simulink model "RGBLEDDimmer_model"  (R2024a)
settings: Solver=FixedStepAuto  StartTime=0.0  StopTime=tFinal  FixedStep=T  RelTol=1e-3  EnableMultiTasking=on
libraries: arduinolib x3, simulink x3
settings Model: SimulationMode=external  ExtModeTrigDuration=2  Creator=Christopher  LastModifiedBy=chris
settings SolverCC: AlgebraicLoopSolver=TrustRegion  AutoInsertRateTranBlk=on
settings DataIOCC: LimitDataPoints=on  StreamToWorkspace=on  ReturnWorkspaceOutputs=off
settings OptimizationCC: LifeSpan=1  MaxStackSize=64
settings DebuggingCC: UnconnectedInputMsg=warning  UnconnectedOutputMsg=warning  UnconnectedLineMsg=warning  AllowSymbolicDim=off  SFUnexpectedBacktrackingDiag=warning  SFNoUnconditionalDefaultTransitionDiag=warning  SFExecutionAtInitializationDiag=none  ArithmeticOperatorsInVariantConditions=warning
settings HardwareCC: ProdBitPerInt=16  ProdBitPerPointer=16  ProdBitPerSizeT=16  ProdBitPerPtrDiffT=16  ProdLargestAtomicFloat=None  ProdWordSize=8  ProdHWDeviceType=Atmel->AVR
settings ModelReferenceCC: EnableRefExpFcnMdlSchedulingChecks=on  PropagateSignalLabelsOutOfModel=off
settings SFSimCC: SimUseLocalCustomCode=off  CustomCodeUndefinedFunction=UseInterfaceOnly
settings RTWCC: Description=Embedded Coder  SystemTargetFile=ert.tlc  HardwareBoard=Arduino Nano 3.0  TemplateMakefile=ert_default_tmf  RTWVerbose=off  RTWUseLocalCustomCode=off  Toolchain=Arduino AVR  BuildConfiguration=Faster Runs  GPUComputeCapability=3.5
settings CodeAppCC: MangleLength=10  StateflowObjectComments=on
settings ERTTargetCC: MultiwordLength=2048  ERTCustomFileBanners=off  SupportContinuousTime=on  SupportNonInlinedSFcns=on  RemoveResetFunc=off  SupportVariableSizeSignals=on  ModelStepFunctionPrototypeControlCompliant=off  ExtMode=on  ExtModeTransport=3  ExtModeStaticAlloc=on  ExtModeAutomaticAllocSize=off  ExtModeStaticAllocSize=250  ExtModeMexFile=ext_xcp  ExtModeMexArgs='127.0.0.1' 0 17725  ExtModeIntrfLevel=Level2 - Open  ERTSrcFileBannerTemplate=codertarget_code_template.cgt  ERTHdrFileBannerTemplate=codertarget_code_template.cgt  ERTDataSrcFileTemplate=codertarget_code_template.cgt  ERTDataHdrFileTemplate=codertarget_code_template.cgt  ConvertIfToSwitch=off  SuppressUnreachableDefaultCases=off
settings ConfigComp: CovMetricSettings=dw  CovSaveCumulativeToWorkspaceVar=on  CovSaveSingleToWorkspaceVar=on  CovExternalEMLEnable=off

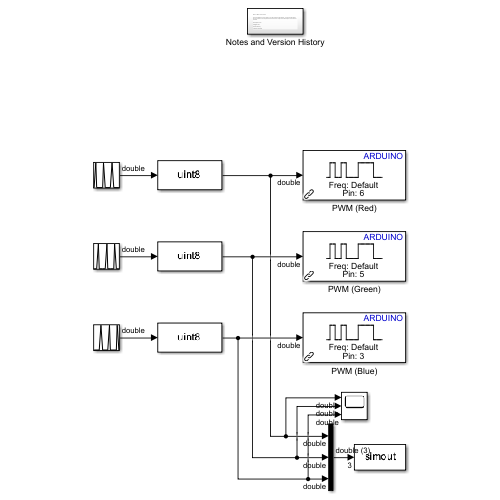
[thumbnail: Simulink's stored preview of the top-level diagram]
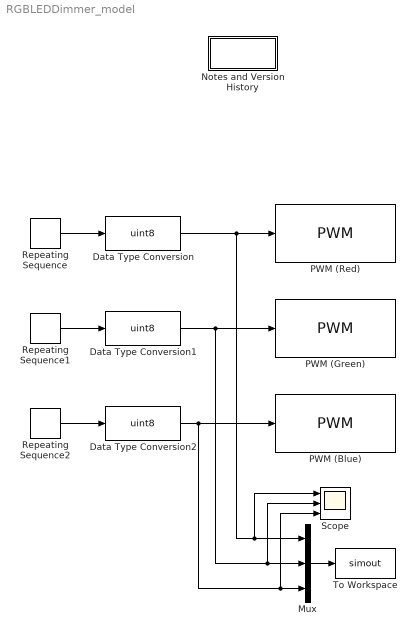
== system RGBLEDDimmer_model ==
  Data Type Conversion : DataTypeConversion  OutDataTypeStr=uint8  SaturateOnIntegerOverflow=off  RndMeth=Floor
  Data Type Conversion1 : DataTypeConversion  OutDataTypeStr=uint8  SaturateOnIntegerOverflow=off  RndMeth=Floor
  Data Type Conversion2 : DataTypeConversion  OutDataTypeStr=uint8  SaturateOnIntegerOverflow=off  RndMeth=Floor
  Mux : Mux  Inputs=3
  Notes and Version History : Subsystem
  PWM (Blue) : arduinolib/PWM  pinNumber=PinLED_B  frequencyType=Default  desiredFrequency=490.2  achievableFrequency=490.2
  PWM (Green) : arduinolib/PWM  pinNumber=PinLED_G  frequencyType=Default  desiredFrequency=490.2  achievableFrequency=490.2
  PWM (Red) : arduinolib/PWM  pinNumber=PinLED_R  frequencyType=Default  desiredFrequency=490.2  achievableFrequency=490.2
  Repeating Sequence : simulink/Sources/Repeating Sequence  rep_seq_t=t_R  rep_seq_y=y_R
  Repeating Sequence1 : simulink/Sources/Repeating Sequence  rep_seq_t=t_G  rep_seq_y=y_G
  Repeating Sequence2 : simulink/Sources/Repeating Sequence  rep_seq_t=t_B  rep_seq_y=y_B
  Scope : Scope  NumInputPorts=3
  To Workspace : ToWorkspace  VariableName=simout  SaveFormat=Structure With Time  SampleTime=-1
  wires:
  Repeating Sequence/1 -> Data Type Conversion/1
  Repeating Sequence1/1 -> Data Type Conversion1/1
  Repeating Sequence2/1 -> Data Type Conversion2/1
  Mux/1 -> To Workspace/1
  Data Type Conversion/1 -> PWM (Red)/1, Scope/1, Mux/1
  Data Type Conversion1/1 -> Scope/2, Mux/2, PWM (Green)/1
  Data Type Conversion2/1 -> Scope/3, Mux/3, PWM (Blue)/1

== system RGBLEDDimmer_model/Notes and Version History ==
  note: Dim 3 LEDs on the board.
      |
      | Use the 'Monitor & Tune' option to run the model on the Arduino. You should be able to see the results on the scope and the result will be output to the Workspace in the simout variable.
      |
      | Christopher Lum
      | lum@uw.edu
      |
      | Version History
      | 12/14/24: Created
